simulink model "sgMdl_IO292_DigitalLoopback"  (R2024b)
settings: Solver=FixedStepAuto  StartTime=0.0  StopTime=inf  RelTol=1e-3  EnableMultiTasking=on
libraries: speedgoatlib_IO292 x3
Description:
  | IO292 - Digital Loopback
settings Model: sg_rtwmakecfg_data=_sglibc__libsg_  ModifiedByFormat=Speedgoat  SimulationMode=external  ExtModeTrigDuration=100000  Creator=Speedgoat  LastModifiedBy=Speedgoat
settings SolverCC: ConcurrentTasks=on  AlgebraicLoopSolver=TrustRegion  PositivePriorityOrder=on  AutoInsertRateTranBlk=on  InsertRTBMode=Never (minimum delay)
settings DataIOCC: SaveFormat=StructureWithTime  ReturnWorkspaceOutputs=off
settings OptimizationCC: BlockReduction=off  OptimizeBlockIOStorage=off  BufferReuse=off  ReuseModelBlockBuffer=off  GlobalBufferReuse=off  ExpressionFolding=off  LocalBlockOutputs=off  OptimizeDataStoreBuffers=off  BusAssignmentInplaceUpdate=off
settings DebuggingCC: TasksWithSamePriorityMsg=none  UnconnectedInputMsg=warning  UnconnectedOutputMsg=warning  UnconnectedLineMsg=warning  ArithmeticOperatorsInVariantConditions=warning
settings HardwareCC: ProdBitPerLong=64  ProdLongLongMode=on  ProdHWDeviceType=Intel->x86-64 (Linux 64)
settings ModelReferenceCC: EnableRefExpFcnMdlSchedulingChecks=on
settings SFSimCC: CustomCodeUndefinedFunction=UseInterfaceOnly
settings RTWCC: Description=Speedgoat Real-Time Target Machine  SystemTargetFile=speedgoat.tlc  TemplateMakefile=slrealtime_default_tmf  Toolchain=Simulink Real-Time Toolchain  BuildConfiguration=Faster Runs  TargetLang=C++  GPUComputeCapability=3.5  DLArmComputeVersion=19.05
settings CodeAppCC: StateflowObjectComments=on
settings SimulinkRealTimeTargetCC: SubcomponentCodeInterfacePackaging=Reusable function  InstructionSetFMA=off  LogToMDFFile=off  SLRTFileLogMaxRuns=10  UseGCCFastMath=on
settings ConfigComp: CovBoundaryAbsTol=1.0e-5

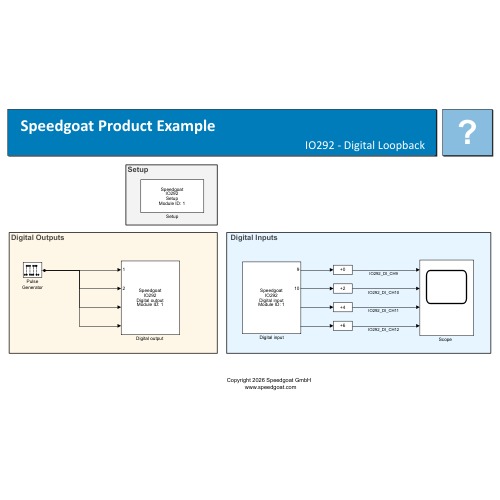
[thumbnail: Simulink's stored preview of the top-level diagram]
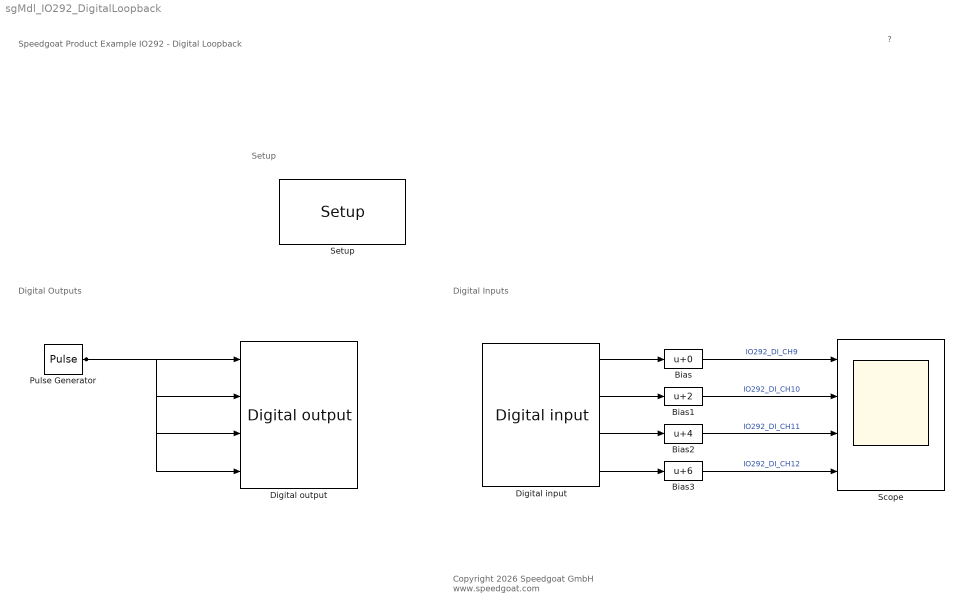
== system sgMdl_IO292_DigitalLoopback ==
  note: Setup
  note: Digital Inputs
  note: Digital Outputs
  note: Speedgoat Product Example
      | IO292 - Digital Loopback
  note: ?
  note: Copyright 2026 Speedgoat GmbH
      |  www.speedgoat.com
  Bias : Bias  SaturateOnIntegerOverflow=off
  Bias1 : Bias  Bias=2  SaturateOnIntegerOverflow=off
  Bias2 : Bias  Bias=4  SaturateOnIntegerOverflow=off
  Bias3 : Bias  Bias=6  SaturateOnIntegerOverflow=off
  Digital input : speedgoatlib_IO292/Digital input   parModuleId=1  parSampleTime=0.001  parPortConf=1 port for each active input channel  parDataType=Double  parPciSlot=-1  parInputChannels=[9 10 11 12]
      settings: SourceProductName=Simulink Real-Time: Speedgoat I/O Blockset
  "Digital output " : speedgoatlib_IO292/Digital output   parModuleId=1  parSampleTime=0.001  parPortConf=1 port for each active output channel  parPciSlot=-1  parOutputChannels=[1 2 3 4]  parOutputInitValues=[0 0 0 0]  parOutputResetValues=[1 1 1 1]
      settings: SourceProductName=Simulink Real-Time: Speedgoat I/O Blockset
  Pulse Generator : DiscretePulseGenerator  Period=200  PulseWidth=100  SampleTime=0.001
  "Scope  " : Scope  NumInputPorts=4
  Setup : speedgoatlib_IO292/Setup   parModuleId=1  parPciSlot=-1  parOutputChannels=[1:4]  parOutputInitValues=0  parOutputResetValues=1  parInputChannels=[9:12]
      settings: SourceProductName=Simulink Real-Time: Speedgoat I/O Blockset
  wires:
  Digital input/1 -> Bias/1
  Digital input/2 -> Bias1/1
  Digital input/3 -> Bias2/1
  Digital input/4 -> Bias3/1
  Pulse Generator/1 -> "Digital output "/4, "Digital output "/3, "Digital output "/2, "Digital output "/1
  Bias/1 -> "Scope  "/1  "IO292_DI_CH9"
  Bias2/1 -> "Scope  "/3  "IO292_DI_CH11"
  Bias3/1 -> "Scope  "/4  "IO292_DI_CH12"
  Bias1/1 -> "Scope  "/2  "IO292_DI_CH10"
